simulink model "discrete_observer"  (R2020b)
settings: Solver=VariableStepAuto  StartTime=0.0  StopTime=10.0  RelTol=1e-3
settings Model: Creator=10853  LastModifiedBy=10853

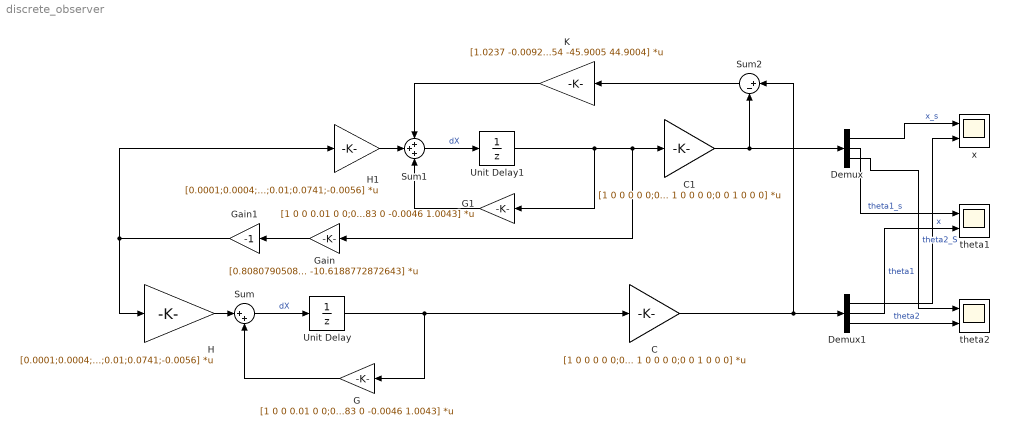
== system discrete_observer ==
  C : Gain  Gain=[1 0 0 0 0 0;0 1 0 0 0 0;0 0 1 0 0 0]  Multiplication=Matrix(K*u)
  C1 : Gain  Gain=[1 0 0 0 0 0;0 1 0 0 0 0;0 0 1 0 0 0]  Multiplication=Matrix(K*u)
  Demux : Demux  Outputs=3
  Demux1 : Demux  Outputs=3
  G : Gain  Gain=[1 0 0 0.01 0 0;0 1.0095 -0.0059 0 0.01 0;0 -0.0046 1.0043 0 0 0.01; 0 0 0 1 0 0;0 1.9009 -1.1747 0 1.0095 -0.0059; 0 -0.9129 0.8583 0 -0.0046 1.0043]  Multiplication=Matrix(K*u)
  G1 : Gain  Gain=[1 0 0 0.01 0 0;0 1.0095 -0.0059 0 0.01 0;0 -0.0046 1.0043 0 0 0.01; 0 0 0 1 0 0;0 1.9009 -1.1747 0 1.0095 -0.0059; 0 -0.9129 0.8583 0 -0.0046 1.0043]  Multiplication=Matrix(K*u)
  Gain : Gain  Gain=[0.808079050860791 100.847272737157 -106.506186957940 1.59703885887324 4.21261961968780 -10.6188772872643]  Multiplication=Matrix(K*u)
  Gain1 : Gain  Gain=-1
  H : Gain  Gain=[0.0001;0.0004;0;0.01;0.0741;-0.0056]  Multiplication=Matrix(K*u)
  H1 : Gain  Gain=[0.0001;0.0004;0;0.01;0.0741;-0.0056]  Multiplication=Matrix(K*u)
  K : Gain  Gain=[1.0237 -0.0092 0.0286; -0.0303 1.6080 -0.5360;0.0030 -0.4498 1.4404;2.3782 -0.9157 2.8586; -3.0631 62.5896 -54.9436; 0.3154 -45.9005 44.9004]  Multiplication=Matrix(K*u)
  Sum : Sum  Inputs=|++
  Sum1 : Sum  Inputs=+++
  Sum2 : Sum  Inputs=|+-
  Unit Delay : UnitDelay  InitialCondition=[0 pi/36 pi/36 0 0 0]  SampleTime=0.01  HasFrameUpgradeWarning=on
  Unit Delay1 : UnitDelay  InitialCondition=[0 0 0 0 0 0]  SampleTime=0.01  HasFrameUpgradeWarning=on
  theta1 : Scope  NumInputPorts=2
  theta2 : Scope  NumInputPorts=2
  x : Scope  NumInputPorts=2
  wires:
  H/1 -> Sum/1
  Sum/1 -> Unit Delay/1  "dX"
  G/1 -> Sum/2
  Unit Delay/1 -> C/1, G/1
  Gain/1 -> Gain1/1
  Gain1/1 -> H1/1, H/1
  Sum1/1 -> Unit Delay1/1  "dX"
  Unit Delay1/1 -> Gain/1, C1/1, G1/1
  C1/1 -> Demux/1, Sum2/2
  C/1 -> Demux1/1, Sum2/1
  G1/1 -> Sum1/3
  H1/1 -> Sum1/2
  Sum2/1 -> K/1
  Demux/2 -> theta1/1  "theta1_s"
  Demux/3 -> theta2/1  "theta2_S"
  Demux1/3 -> theta2/2  "theta2"
  K/1 -> Sum1/1
  Demux/1 -> x/1  "x_s"
  Demux1/1 -> x/2  "x"
  Demux1/2 -> theta1/2  "theta1"
